simulink model "FORWARD_KINEMATICS"  (R2019b)
settings: Solver=VariableStepAuto  StartTime=0.0  StopTime=6  MaxStep=0.01  MinStep=0.01  RelTol=1e-3  EnableMultiTasking=on
model workspace: external: MATLAB File D:\Google Drive\Duongw_Folder\Thesis Master\_Model\Delta_Model_ADEPT\SIMCAPE_MULTI_BODY\ADEPT_DELTA_3AXES1\Assem1_ADEPT_HORNET_DataFile.m (data not in the file)
values from neighbouring files (symbols this model uses):
  l1 = 0.315    [Assem1_ADEPT_HORNET_DataFile.m]    (also in LinePath_Inverse_Dynamic_Model.m; Plot_Forward_trajectory_PD_controller.m; UPath_Inverse_Dynamic_Model.m; data_kinematicDimension.m)
  phi = [1.5707963267948966; 3.6651914291880918; 5.7595865315812871]    [Assem1_ADEPT_HORNET_DataFile.m]    (also in LinePath_Inverse_Dynamic_Model.m = [phi1; phi2; phi3]; Plot_Forward_trajectory_PD_controller.m = [phi1; phi2; phi3]; UPath_Inverse_Dynamic_Model.m = [phi1; phi2; phi3]; data_kinematicDimension.m = [phi1; phi2; phi3])
  r = 0.15000000000000002    (= 0.15)    [Assem1_ADEPT_HORNET_DataFile.m]    (also in LinePath_Inverse_Dynamic_Model.m = -0.15; Plot_Forward_trajectory_PD_controller.m; UPath_Inverse_Dynamic_Model.m = -0.15; data_kinematicDimension.m)
settings Model: Creator=computer  LastModifiedBy=ShiningDanyang
settings DataIOCC: SaveFormat=Array  ReturnWorkspaceOutputs=off
settings OptimizationCC: LifeSpan=inf
settings DebuggingCC: SFUnexpectedBacktrackingDiag=warning  SFNoUnconditionalDefaultTransitionDiag=warning  SFExecutionAtInitializationDiag=none  ArithmeticOperatorsInVariantConditions=warning
settings SFSimCC: SimUseLocalCustomCode=off  CustomCodeUndefinedFunction=UseInterfaceOnly
settings RTWCC: RTWUseLocalCustomCode=off
settings CodeAppCC: StateflowObjectComments=on
settings GRTTargetCC: TargetLangStandard=C89/C90 (ANSI)  GeneratePreprocessorConditionals=Disable all
settings ConfigComp: CovMetricSettings=dw  CovHtmlReporting=on  CovSaveCumulativeToWorkspaceVar=on  CovSaveSingleToWorkspaceVar=on  CovExternalEMLEnable=off

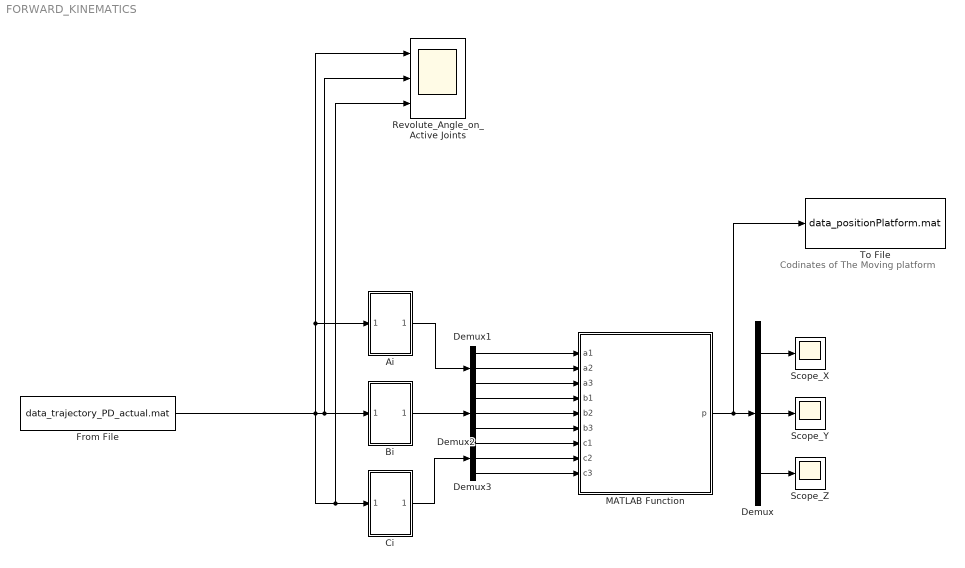
== system FORWARD_KINEMATICS ==
  note: Codinates of The Moving platform
  Ai : Subsystem
  Bi : Subsystem
  Ci : Subsystem
  Demux{,1..3} (4 alike) : Demux  Outputs=3
  From File : FromFile  FileName=data_trajectory_PD_actual.mat  SampleTime=0  InterpolationWithinTimeRange=Zero order hold
  MATLAB Function : MATLAB Function  TreatAsAtomicUnit=on
  Revolute_Angle_on_Active Joints : Scope  NumInputPorts=3
  Scope_X : Scope
  Scope_Y : Scope
  Scope_Z : Scope
  To File : ToFile  Filename=data_positionPlatform.mat  MatrixName=xyz
  wires:
  Demux/3 -> Scope_Z/1
  Demux/2 -> Scope_Y/1
  Demux/1 -> Scope_X/1
  MATLAB Function/1(p) -> To File/1, Demux/1
  Bi/1(Out1) -> Demux2/1
  Demux3/2 -> MATLAB Function/8(c2)
  Demux3/1 -> MATLAB Function/7(c1)
  From File/1 -> Ai/1(In1), Revolute_Angle_on_Active Joints/1, Revolute_Angle_on_Active Joints/3, Ci/1(In1), Bi/1(In1), Revolute_Angle_on_Active Joints/2
  Demux3/3 -> MATLAB Function/9(c3)
  Demux2/1 -> MATLAB Function/4(b1)
  Demux2/3 -> MATLAB Function/6(b3)
  Ai/1(Out1) -> Demux1/1
  Demux2/2 -> MATLAB Function/5(b2)
  Ci/1(Out1) -> Demux3/1
  Demux1/2 -> MATLAB Function/2(a2)
  Demux1/1 -> MATLAB Function/1(a1)
  Demux1/3 -> MATLAB Function/3(a3)

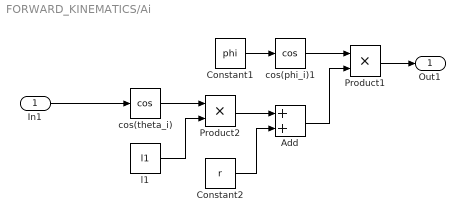
== system FORWARD_KINEMATICS/Ai ==
  In1 : Inport
  Add : Sum
  Constant1 : Constant  Value=phi
  Constant2 : Constant  Value=r
  Product1 : Product
  Product2 : Product
  cos(phi_i)1 : Trigonometry  Operator=cos
  cos(theta_i) : Trigonometry  Operator=cos
  l1 : Constant  Value=l1
  Out1 : Outport  VectorParamsAs1DForOutWhenUnconnected=off
  wires:
  Constant1/1 -> cos(phi_i)1/1
  cos(theta_i)/1 -> Product2/1
  In1/1 -> cos(theta_i)/1
  l1/1 -> Product2/2
  cos(phi_i)1/1 -> Product1/1
  Product2/1 -> Add/1
  Constant2/1 -> Add/2
  Add/1 -> Product1/2
  Product1/1 -> Out1/1

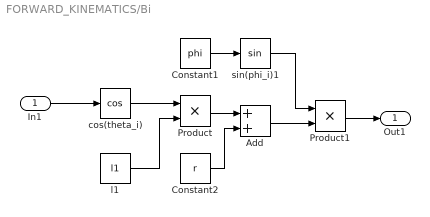
== system FORWARD_KINEMATICS/Bi ==
  In1 : Inport
  Add : Sum
  Constant1 : Constant  Value=phi
  Constant2 : Constant  Value=r
  Product : Product
  Product1 : Product
  cos(theta_i) : Trigonometry  Operator=cos
  l1 : Constant  Value=l1
  sin(phi_i)1 : Trigonometry
  Out1 : Outport  VectorParamsAs1DForOutWhenUnconnected=off
  wires:
  In1/1 -> cos(theta_i)/1
  l1/1 -> Product/2
  cos(theta_i)/1 -> Product/1
  Constant1/1 -> sin(phi_i)1/1
  Product/1 -> Add/1
  Constant2/1 -> Add/2
  Add/1 -> Product1/2
  sin(phi_i)1/1 -> Product1/1
  Product1/1 -> Out1/1

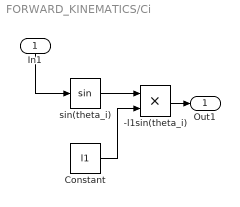
== system FORWARD_KINEMATICS/Ci ==
  In1 : Inport
  -l1sin(theta_i) : Product
  Constant : Constant  Value=l1
  sin(theta_i) : Trigonometry
  Out1 : Outport  VectorParamsAs1DForOutWhenUnconnected=off
  wires:
  Constant/1 -> -l1sin(theta_i)/2
  In1/1 -> sin(theta_i)/1
  -l1sin(theta_i)/1 -> Out1/1
  sin(theta_i)/1 -> -l1sin(theta_i)/1

== matlab function FORWARD_KINEMATICS/MATLAB Function ==
  data: p output; a1 input; a2 input; a3 input; b1 input; b2 input; b3 input; c1 input; c2 input; c3 input
function p = equasol(a1, a2, a3, b1, b2, b3, c1, c2, c3)
%#codegen
 coder.extrinsic('solequa'); 
 p = zeros(3,1);
 p = solequa(a1, a2, a3, b1, b2, b3, c1, c2, c3);
